simulink model "Throttle_Dyno_V3"  (R2022b)
settings: Solver=FixedStepAuto  StartTime=0.0  StopTime=10000.0  FixedStep=.01  RelTol=1e-3  EnableMultiTasking=on
libraries: canmsglib x2, raspberrypiCommlib x2, slpidlib x1
settings Model: Creator=david  LastModifiedBy=david
settings SolverCC: PositivePriorityOrder=on
settings OptimizationCC: EnhancedBackFolding=on  PassReuseOutputArgsAs=Individual arguments  ZeroExternalMemoryAtStartup=off  ZeroInternalMemoryAtStartup=off  MaxStackSize=64  OptimizeBlockOrder=speed  DifferentSizesBufferReuse=on  OptimizationCustomize=off  EfficientTunableParamExpr=on
settings DebuggingCC: ParameterTunabilityLossMsg=error
settings HardwareCC: ProdBitPerPointer=32  ProdBitPerSizeT=32  ProdBitPerPtrDiffT=32  ProdLargestAtomicInteger=Long  ProdLargestAtomicFloat=Double  ProdWordSize=32  ProdLongLongMode=on  ProdHWDeviceType=ARM Compatible->ARM Cortex
settings RTWCC: Description=Embedded Coder  SystemTargetFile=ert.tlc  HardwareBoard=Raspberry Pi  TLCOptions="-aInlineSetEventsForThisBaseRateFcn=TLC_FALSE -aSuppressMultiTaskScheduler=TLC_FALSE  -aRateBasedStepFcn=0"  TemplateMakefile=ert_default_tmf  Toolchain=GNU GCC Embedded Linux  BuildConfiguration=Faster Runs
settings CodeAppCC: ForceParamTrailComments=on  IgnoreCustomStorageClasses=off  OperatorAnnotations=on  SimulinkDataObjDesc=on  SFDataObjDesc=on  InsertBlockDesc=on
settings ERTTargetCC: SupportVariableSizeSignals=on  ExtModeTransport=2  ExtModeStaticAlloc=on  ExtModeMexFile=ext_xcp  ExtModeIntrfLevel=Level2 - Open

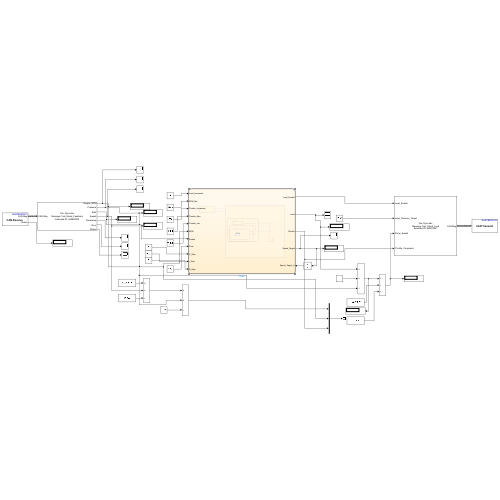
[thumbnail: Simulink's stored preview of the top-level diagram]
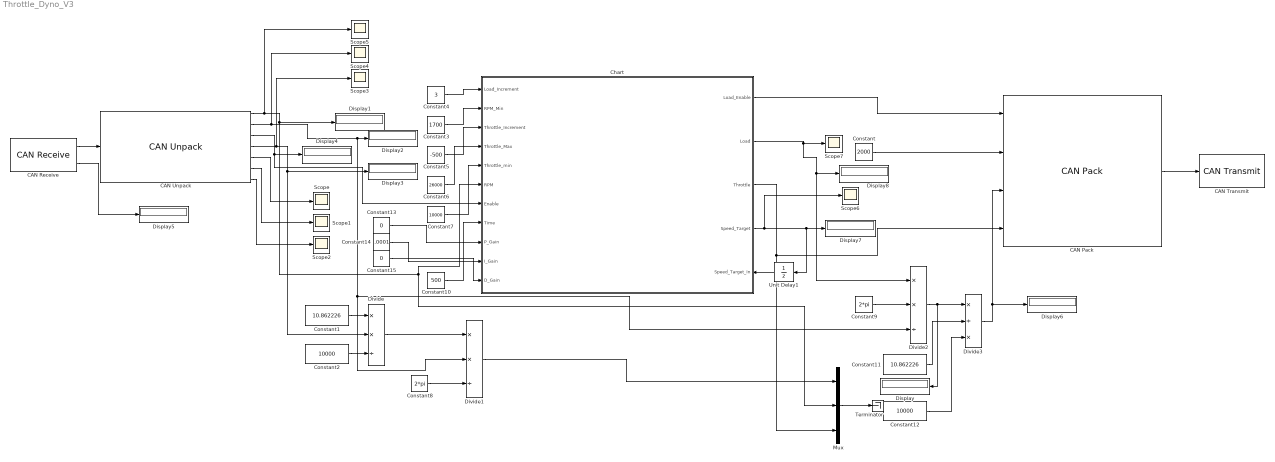
== system Throttle_Dyno_V3 ==
  CAN Pack : canmsglib/CAN Pack  CANdbFile=C:\Git\2023_Tractor_Plant_Models\Dyno.dbc  MsgList=Test_Stand_Load  MsgName=Test_Stand_Load  MsgIDType=Extended (29-bit identifier)  MsgIdentifier=469827841  MsgLength=8  Remote=off  ApplyMinMax=off  BusOutput=on  SignalInfo={'Load_Enable','63','1','LE','unsigned','Standard','0','1','0','0','1';'Load_Pressure_Target','0','16','LE','unsigned','Standard','0','1','0','0','3500';'Pump_Swash','16','16','LE','unsigned','Standard','0','1','0','0','10000';'Throttle_Command','40','16','LE','unsigned','Standard','0','1','0','0','26000'}
      settings: LibrarySourceBlock=embeddedtargetslib/Host Communication/CAN Pack  DataFormat=CANdb specified signals
  CAN Receive : raspberrypiCommlib/CAN Receive  DeviceID=can0  SetupCAN=off  TypeofCAN=Real  OutputDataType=CAN Msg  IdentifierType=Standard (11-bit identifier)  MessageId=100  MsgLength=8  SampleTime=.01  OutputError=off  OutputRemote=off  SimulateUsing=Code generation
  CAN Transmit : raspberrypiCommlib/CAN Transmit  DeviceID=can0  SetupCAN=off  TypeofCAN=Real  InputDataType=CAN Msg  BlockingMode_=off  BlockTimeout_=1  OutputStatus=off  IdentifierType=Standard (11-bit identifier)  MessageId=100  MsgLength=8  RemoteFrame=off  SimulateUsing=Code generation
  CAN Unpack : canmsglib/CAN Unpack  CANdbFile=C:\Git\2023_Tractor_Plant_Models\Dyno.dbc  MsgList=Test_Stand_Feedback  MsgName=Test_Stand_Feedback  MsgIDType=Extended (29-bit identifier)  MsgIdentifier=469828098  MsgLength=8  SignalInfo={'Engine_RPM','0','16','LE','unsigned','Standard','0','1','0','0','3800';'Pressure','16','16','LE','unsigned','Standard','0','1','0','0','5000';'Start','48','1','LE','unsigned','Standard','0','1','0','0','1';'Swash','32','16','LE','unsigned','Standard','0','1','0','0','10000'}  IDPort=off  TimestampPort=on  ErrorPort=on  RemotePort=off  LengthPort=off  StatusPort=on  ApplyMinMax=off
      settings: LibrarySourceBlock=embeddedtargetslib/Host Communication/CAN Unpack  DataFormat=CANdb specified signals
  Chart : Stateflow chart  TreatAsAtomicUnit=on
      settings: PortSchema="{\"entries\":[{\"content\":{\"sides\":[{\"content\":{\"connectorIds\":[\"In1\",\"In2\",\"In3\",\"In4\",\"In5\",\"In6\",\"In7\",\"In8\",\"In9\",\"In10\",\"In11\"]},\"type\":\"ConnectorPlacement.EquallySpacedRectSide\",\"uuid\":\"232d95f6-ea30-407d-a8dc-544f3f699a84\"},{\"content\":{\"connectorIds\":[\"Out1\",\"Out2\",\"Out3\",\"Out4\",\"In12\"],\"side\":\"RIGHT\"},\"type\":\"ConnectorPlacement.EquallySpacedRectSide\",\"uuid\":\"6d17f04d-0cb7-478e-b8f1-d994f7d5a903\"},{\"content\":{\"connectorIds\":[],\"side\":\"TOP\"},\"type\":\"ConnectorPlacement.EquallySpacedRectSide\",\"uuid\":\"782bd91f-32be-4e92-9e22-b96eff913ffc\"}]},\"type\":\"ConnectorPlacement.EquallySpacedConnector\",\"uuid\":\"ed86112d-d962-4886-8e77-9225cf3002e5\"}],\"packageUris\":[\"http://schema.mathworks.com/mf0/Connector/R2020b\"],\"version\":\"1.0\"}"
  Constant : Constant  Value=2000
  Constant1 : Constant  Value=10.862226
  Constant10 : Constant  Value=500
  Constant11 : Constant  Value=10.862226
  Constant12 : Constant  Value=10000
  Constant13 : Constant  Value=0
  Constant14 : Constant  Value=.0001
  Constant15 : Constant  Value=0
  Constant2 : Constant  Value=10000
  Constant3 : Constant  Value=1700
  Constant4 : Constant  Value=3
  Constant5 : Constant  Value=-500
  Constant6 : Constant  Value=26000
  Constant7 : Constant  Value=10000
  Constant8 : Constant  Value=2*pi
  Constant9 : Constant  Value=2*pi
  Display{,1..8} (9 alike) : Display
  Divide : Product  Inputs=**/
  Divide1 : Product  Inputs=**/
  Divide2 : Product  Inputs=**/
  Divide3 : Product  Inputs=*/*
  Mux : Mux  Inputs=3
  Scope{,1..7} (8 alike) : Scope
  Terminator : Terminator
  Unit Delay1 : UnitDelay  SampleTime=-1  HasFrameUpgradeWarning=on
  wires:
  CAN Unpack/3 -> Display4/1, Chart/7(Enable)
  Mux/1 -> Terminator/1
  CAN Unpack/2 -> Scope4/1, Display2/1, Divide2/3, Divide1/2
  Chart/1(Load_Enable) -> CAN Pack/1
  Constant4/1 -> Chart/1(Load_Increment)
  Constant/1 -> CAN Pack/2
  Constant5/1 -> Chart/3(Throttle_Increment)
  Constant3/1 -> Chart/2(RPM_Min)
  CAN Unpack/1 -> Scope5/1, Display1/1, Mux/2, Chart/6(RPM)
  Divide/1 -> Divide1/1
  CAN Pack/1 -> CAN Transmit/1
  Constant2/1 -> Divide/3
  CAN Unpack/4 -> Scope3/1, Display3/1, Divide/2
  Constant7/1 -> Chart/5(Throttle_min)
  Chart/3(Throttle) -> Mux/3, CAN Pack/4
  Constant6/1 -> Chart/4(Throttle_Max)
  Constant1/1 -> Divide/1
  Constant8/1 -> Divide1/3
  CAN Receive/1 -> CAN Unpack/1
  CAN Receive/2 -> Display5/1
  Divide1/1 -> Mux/1
  Constant9/1 -> Divide2/2
  Chart/2(Load) -> Display8/1, Divide2/1, Scope7/1
  Divide2/1 -> Display/1, Divide3/1
  Constant11/1 -> Divide3/2
  Constant12/1 -> Divide3/3
  Divide3/1 -> Display6/1, CAN Pack/3
  Constant10/1 -> Chart/8(Time)
  CAN Unpack/5 -> Scope/1
  CAN Unpack/6 -> Scope1/1
  CAN Unpack/7 -> Scope2/1
  Chart/4(Speed_Target) -> Unit Delay1/1, Display7/1, Scope6/1
  Constant13/1 -> Chart/9(P_Gain)
  Constant14/1 -> Chart/10(I_Gain)
  Constant15/1 -> Chart/11(D_Gain)
  Unit Delay1/1 -> Chart/12(Speed_Target_In)

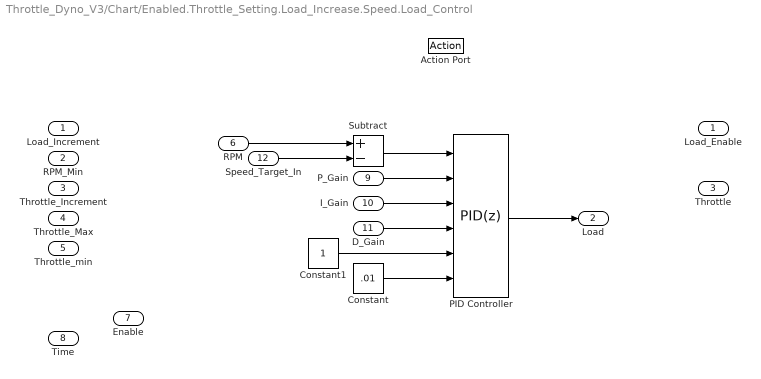
== system Throttle_Dyno_V3/Chart/Enabled.Throttle_Setting.Load_Increase.Speed.Load_Control ==
  Load_Increment : Inport
  RPM_Min : Inport  Port=2
  Throttle_Increment : Inport  Port=3
  Throttle_Max : Inport  Port=4
  Throttle_min : Inport  Port=5
  RPM : Inport  Port=6
  Enable : Inport  Port=7
  Time : Inport  Port=8
  P_Gain : Inport  Port=9
  I_Gain : Inport  Port=10
  D_Gain : Inport  Port=11
  Speed_Target_In : Inport  Port=12
  Action Port : ActionPort
      settings: CopyFcn=Stateflow.SLINSF.SimulinkMan.removeBlockPreDeleteFcn  PreDeleteFcn=Stateflow.SLINSF.SimulinkMan.unsafePredeleteFcn
  Constant : Constant  Value=.01
  Constant1 : Constant
  PID Controller : slpidlib/PID Controller  Controller=PID  Form=Parallel  TimeDomain=Discrete-time  UseExternalTs=on  SampleTime=-1  IntegratorMethod=Forward Euler  FilterMethod=Forward Euler  ControllerParametersSource=external  P=1  I=1  UseKiTs=off  D=0  N=100  UseFilter=on  TunerSelectOption=Transfer Function Based (PID Tuner App)  InitialConditionSource=internal  InitialConditionForIntegrator=0  InitialConditionForFilter=0  DifferentiatorICPrevScaledInput=0  ExternalReset=none  TrackingMode=off  Kt=1  LimitOutput=off  SatLimitsSource=internal  UpperSaturationLimit=inf  LowerSaturationLimit=-inf  LinearizeAsGain=on  AntiWindupMode=none  Kb=1  LimitIntegrator=off  UpperIntegratorSaturationLimit=inf  LowerIntegratorSaturationLimit=-inf  POutMin=[]  POutMax=[]  IOutMin=[]  IOutMax=[]  DOutMin=[]  DOutMax=[]  NOutMin=[]  NOutMax=[]  SumOutMin=[]  SumOutMax=[]  SaturationOutMin=[]  SaturationOutMax=[]  PParamMin=[]  PParamMax=[]  IParamMin=[]  IParamMax=[]  DParamMin=[]  DParamMax=[]  NParamMin=[]  NParamMax=[]  KbParamMin=[]  KbParamMax=[]  KtParamMin=[]  KtParamMax=[]  KbOutMin=[]  KbOutMax=[]  KtOutMin=[]  KtOutMax=[]  IntegratorOutMin=[]  IntegratorOutMax=[]  FilterOutMin=[]  FilterOutMax=[]  SumI1OutMin=[]  SumI1OutMax=[]  SumI2OutMin=[]  SumI2OutMax=[]  SumI3OutMin=[]  SumI3OutMax=[]  SumI4OutMin=[]  SumI4OutMax=[]  SumDOutMin=[]  SumDOutMax=[]  DifferentiatorOutMin=[]  DifferentiatorOutMax=[]  FilterDiffOutCoefMin=[]  FilterDiffOutCoefMax=[]  ReciprocalOutMin=[]  ReciprocalOutMax=[]  SumDenOutMin=[]  SumDenOutMax=[]  SumNumOutMin=[]  SumNumOutMax=[]  DivideOutMin=[]  DivideOutMax=[]  UdiffTsProdOutMin=[]  UdiffTsProdOutMax=[]  NTsProdOutMin=[]  NTsProdOutMax=[]  UintegralTsProdOutMin=[]  UintegralTsProdOutMax=[]  UngainTsProdOutMin=[]  UngainTsProdOutMax=[]  ClampingZeroOutDataTypeStr=Inherit: Inherit via back propagation  ClampingZeroOutMin=[]  ClampingZeroOutMax=[]  FilterDenConstantOutDataTypeStr=Inherit: Inherit via back propagation  FilterDenConstantOutMin=[]  FilterDenConstantOutMax=[]  PCopyOutDataTypeStr=Inherit: Inherit via back propagation  PCopyOutMin=[]  PCopyOutMax=[]  NCopyOutDataTypeStr=Inherit: Inherit via back propagation  NCopyOutMin=[]  NCopyOutMax=[]  IntegratorContinuousStateAttributes=''  IntegratorStateMustResolveToSignalObject=off  IntegratorRTWStateStorageClass=Auto  FilterContinuousStateAttributes=''  FilterStateMustResolveToSignalObject=off  FilterRTWStateStorageClass=Auto  ParallelPVariant=ExternalParameters  IdealPVariant=Disabled  IVariant=ExternalParameters  DVariant=ExternalParameters  IntegratorVariant=Discrete  SatVariant=Disabled  AWVariant=Passthrough  PCopyVariant=Disabled  TRVariant=Disabled  FdbkBlocksVariant=Forward  IdealPFdbkVariant=Disabled  SatFdbkVariant=Disabled  DerivativeFilterVariant=ForwardEulerFilter  NVariant=ExternalParameters  NCopyVariant=Disabled  FilterICVariant=InternalICsFilter  IntegratorICVariant=InternalICs  ExternalResetVariant=Disabled  TRSumVariant=Passthrough  SumFdbkVariant=Disabled  SumVariant=Sum_PID  TsampFilterVariant=ExternalTs  TsampNgainVariant=ExternalTs  TsampIntegralVariant=ExternalTs  ExternalSaturationOutDataTypeStr=Inherit: Same as second input
  Subtract : Sum  Inputs=+-
  Load_Enable : Outport
  Load : Outport  Port=2
  Throttle : Outport  Port=3
  wires:
  Speed_Target_In/1 -> Subtract/2
  Subtract/1 -> PID Controller/1
  P_Gain/1 -> PID Controller/2
  I_Gain/1 -> PID Controller/3
  D_Gain/1 -> PID Controller/4
  Constant/1 -> PID Controller/6
  Constant1/1 -> PID Controller/5
  PID Controller/1 -> Load/1
  RPM/1 -> Subtract/1

== stateflow chart Throttle_Dyno_V3/Chart ==
  state Enabled
    state Throttle_Setting
      en:
      state Start
        en:
        Load_Enable=true;
        Load=0;
      state Load_Increase
        en:
        Speed_Target=RPM-200;
        state Speed
          state Load_Control
          (default) -> Load_Control : {Load=0}
        (default) -> Speed
        Speed -> (junction 74) : [duration((RPM>Speed_Target-30&&RPM<Speed_Target+30),msec)>3000]
        (junction 74) -> (junction 76)
        (junction 76) -> Speed : {Speed_Target=Speed_Target-50}
      (default) -> Start : {Count=0}
      (junction 21) -> Start : {Count=Count+1}
      (junction 20) -> (junction 21)
      Start -> Load_Increase
      Load_Increase -> (junction 20) : [Speed_Target<=RPM_Min]
    state End
      en,du:
      Throttle=Throttle_min;
      Load=0;
      Load_Enable=false;
    (default) -> Throttle_Setting
    (junction 28) -> Throttle_Setting : {Count=0}
    (junction 26) -> (junction 28) [order 2] : {Throttle=Throttle+Throttle_Increment}
    Throttle_Setting -> (junction 26) : [Count==2]
    (junction 26) -> End [order 1] : [Throttle<=Throttle_min]
  state Disabled
    en,du:
    Load_Enable=false;
    Load=0;
    Throttle=Throttle_Max;
  (default) -> Disabled
  Disabled -> Enabled : [hasChangedTo(Enable,true)]
  Enabled -> Disabled : [~Enable]
  data: sf_internal_action_state_placeholder_data local double size=1 =0; Load_Increment input; RPM_Min input; Throttle_Increment input; Throttle_Max input; Throttle_min input; Load_Enable output; Count local; Load output; Throttle output; RPM input; Enable input; Time input; P_Gain input; I_Gain input; D_Gain input; Speed_Target_In input; Speed_Target output =3600
